simulink model "mconversionBus1"  (Simulink 8.0)
settings: Solver=ode3  StartTime=0.0  StopTime=10.0  RelTol=1e-3
settings Model: Creator=awarlock  LastModifiedBy=htu  ExtModeAutoUpdateStatusClock=off
settings DataIOCC: SignalLoggingSaveFormat=ModelDataLogs
settings OptimizationCC: InlineParams=on  InlineInvariantSignals=on  InitFltsAndDblsToZero=on
settings DebuggingCC: SaveWithParameterizedLinksMsg=none  SignalResolutionControl=TryResolveAllWithWarning  MultiTaskDSMMsg=warning  MultiTaskCondExecSysMsg=none
settings RTWCC: IncludeERTFirstTime=on
settings GRTTargetCC: TargetFcnLib=ansi_tfl_tmw.mat  CombineOutputUpdateFcns=off  GRTInterface=on

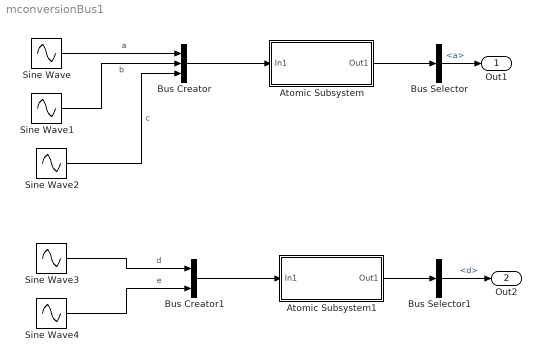
== system mconversionBus1 ==
  Atomic Subsystem : Subsystem  TreatAsAtomicUnit=on
  Atomic Subsystem1 : Subsystem  TreatAsAtomicUnit=on
  Bus Creator : BusCreator  DialogController=Simulink.DDGSource_Bus  Inputs=3
  Bus Creator1 : BusCreator  DialogController=Simulink.DDGSource_Bus  Inputs=2
  Bus Selector : BusSelector  DialogController=Simulink.DDGSource_Bus  OutputSignals=a
  Bus Selector1 : BusSelector  DialogController=Simulink.DDGSource_Bus  OutputSignals=d
  Sine Wave{,1..4} (5 alike) : Sin  SampleTime=0.1
  Out1 : Outport
  Out2 : Outport  Port=2
  wires:
  Bus Creator/1 -> Atomic Subsystem/1(In1)
  Bus Creator1/1 -> Atomic Subsystem1/1(In1)
  Atomic Subsystem/1(Out1) -> Bus Selector/1
  Atomic Subsystem1/1(Out1) -> Bus Selector1/1
  Sine Wave/1 -> Bus Creator/1  "a"
  Sine Wave1/1 -> Bus Creator/2  "b"
  Sine Wave2/1 -> Bus Creator/3  "c"
  Sine Wave3/1 -> Bus Creator1/1  "d"
  Sine Wave4/1 -> Bus Creator1/2  "e"
  Bus Selector/1 -> Out1/1  "<a>"
  Bus Selector1/1 -> Out2/1  "<d>"

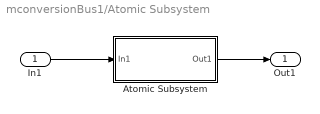
== system mconversionBus1/Atomic Subsystem ==
  In1 : Inport
  Atomic Subsystem : Subsystem  TreatAsAtomicUnit=on
  Out1 : Outport
  wires:
  In1/1 -> Atomic Subsystem/1(In1)
  Atomic Subsystem/1(Out1) -> Out1/1

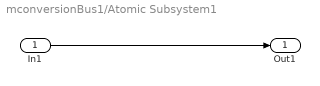
== system mconversionBus1/Atomic Subsystem1 ==
  In1 : Inport
  Out1 : Outport
  wires:
  In1/1 -> Out1/1

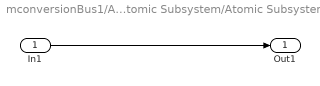
== system mconversionBus1/Atomic Subsystem/Atomic Subsystem ==
  In1 : Inport
  Out1 : Outport
  wires:
  In1/1 -> Out1/1
